simulink model "FSFstatespace"  (R2023b)
settings: Solver=FixedStepAuto  StartTime=0.0  StopTime=10.0  FixedStep=0.01  RelTol=1e-3
undefined symbols (not defined in the file): A, B, C, D, K_real
settings Model: Creator=lxy18  LastModifiedBy=lxy18

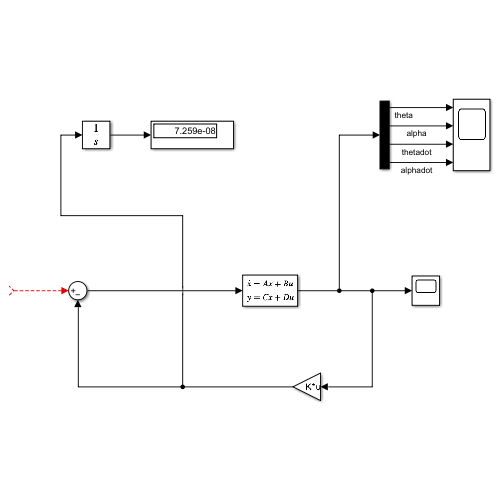
[thumbnail: Simulink's stored preview of the top-level diagram]
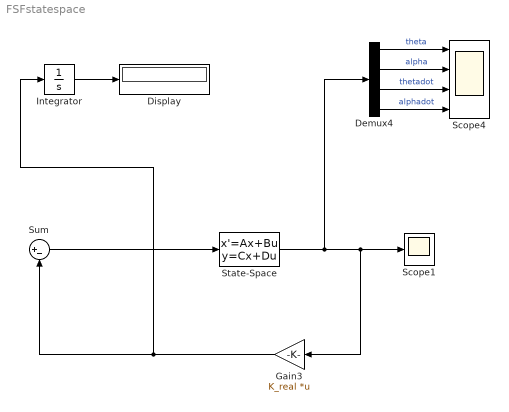
== system FSFstatespace ==
  Demux4 : Demux
  Display : Display
  Gain3 : Gain  Gain=K_real  Multiplication=Matrix(K*u)
  Integrator : Integrator
  Scope1 : Scope
  Scope4 : Scope  NumInputPorts=4
  State-Space : StateSpace  A=A  B=B  C=C  D=D  InitialCondition=[1 * pi / 180; 1 * pi / 180; 0; 0]
  Sum : Sum  Inputs=|+-
  wires:
  Demux4/4 -> Scope4/4  "alphadot"
  Demux4/2 -> Scope4/2  "alpha"
  Demux4/3 -> Scope4/3  "thetadot"
  State-Space/1 -> Gain3/1, Scope1/1, Demux4/1
  Demux4/1 -> Scope4/1  "theta"
  Sum/1 -> State-Space/1
  Gain3/1 -> Integrator/1, Sum/2
  ? -> Sum/1
  Integrator/1 -> Display/1
